simulink model "IEEE34bus_v2019b_Phasor_PI_ZIPload"  (R2024a)
settings: Solver=ode4  StartTime=0.0  StopTime=100  FixedStep=Ts  MaxStep=1e-4  RelTol=1e-4
InitFcn:
  | a=1; % Loading Factor
  | Ts=0.1;% For Delay Blocks in Voltage Regulator Controls
  | % phase to sequence conversion of RXB matrices
  | c=1*exp(sqrt(-1)*(120*pi/180));
  | T=[1 1 1;1 c*c c;1 c c*c];
  | Tinv=1/3*[1 1 1;1 c c*c;1 c*c c];
  | 
  | % Simulation data for the IEEE 34 Node Test Feeder model
  | mi2km = 1.60934;%  miles to km conversion
  | ft2km = 0.0003048; % feet to km conversion
  | ms2F = 1*1e-6/(2*pi*60);% microsiemens to Farads conversion
  | 
  | %% Configuration 300 - series reactance - ohm/mile
  | R_300 = [1.3368 0.2101 0.2130;0.2101 1.3238 0.2066;0.2130 0.2066 1.3294];
  | X_300 = [1.3343 0.5779 0.5015;0.5779 1.3569 0.4591;0.5015 0.4591 1.3471];
  | % charging susceptance - microsiemens/mile
  | B_300 = [5.3350 -1.5313 -0.9943;-1.5313 5.0979 -0.6212;-0.9943 -0.6212 4.8880];
  | 
  | R_300 = R_300/mi2km;
  | Rseq=Tinv*R_300*T;
  | R1_300=Rseq(2,2);R0_300=Rseq(1,1);
  | 
  | L_300 = (X_300/(2*pi*60))/mi2km;
  | Lseq=Tinv*L_300*T;
  | L1_300=Lseq(2,2);L0_300=Lseq(1,1);
  | 
  | C_300 =(B_300*ms2F)/mi2km;
  | Cseq=Tinv*C_300*T;
  | C1_300=Cseq(2,2);C0_300=Cseq(1,1);
  | 
  | %% Configuration 301 - series reactance - ohm/mile
  | R_301 = [1.9300 0.2327 0.2359;0.2327 1.9157 0.2288;0.2359 0.2288 1.9219];
  | X_301 = [1.4115 0.6442 0.5691;0.6442 1.4281 0.5238;0.5691 0.5238 1.4209];
  | % charging susceptance - microsiemens/mile
  | B_301 = [5.1207 -1.4364 -0.9402;-1.4364 4.9055 -0.5951;-0.9402 -0.5951 4.7154];
  | 
  | R_301 = R_301/mi2km;
  | Rseq=Tinv*R_301*T;
  | R1_301=Rseq(2,2);R0_301=Rseq(1,1);
  | 
  | L_301 = (X_301/(2*pi*60))/mi2km;
  | Lseq=Tinv*L_301*T;
  | L1_301=Lseq(2,2);L0_301=Lseq(1,1);
  | 
  | C_301 =(B_301*ms2F)/mi2km;
  | Cseq=Tinv*C_301*T;
  | C1_301=Cseq(2,2);C0_301=Cseq(1,1);
  | 
  | %% Configuration 302 - series reactance - ohm/mile
  | R_302 = [2.7995 0 0;0 0 0;0 0 0];
  | X_302 = [1.4855 0 0;0 0 0;0 0 0];
  | % charging susceptance - microsiemens/mile
  | B_302 = [4.2251 0 0;0 0 0;0 0 0];
  | 
  | R_302 = R_302/mi2km;
  | Rseq=Tinv*R_302*T;
  | R1_302=Rseq(2,2);R0_302=Rseq(1,1);
  | 
  | L_302 = (X_302/(2*pi*60))/mi2km;
  | Lseq=Tinv*L_302*T;
  | ... (+41 lines)
undefined symbols (not defined in the file): find_system, j
libraries: spsSeriesRLCBranchLib x157, spsGroundLib x103, spsVoltageMeasurementLib x100, spsControlledCurrentSourceLib x94, spsThreePhaseVIMeasurementLib x37, spsThreePhasePISectionLineLib x20, spsCurrentMeasurementLib x12, spsOnDelayLib x12, spsPiSectionLineLib x8, spsControlledVoltageSourceLib x6, spsDiscreteVariableTimeDelayLib x6, spsMutualInductanceLib x4
(part 7 of 8)

== system IEEE34bus_v2019b_Phasor_PI_ZIPload/Regulator 2/Single Phase SVR_B/Voltage Regulator Control/Tap Changer Control/Edge Detector ==
  note: Edge or Slope Detector
  In : Inport
  Constant1 : Constant  Value=model
  Demux : Demux  Outputs=2
      settings: DisplayOption=none
  Logical Operator1 : Logic  Operator=OR
  Memory : Memory  InitialCondition=ic  LinearizeAsDelay=on
  Multiport Switch : MultiPortSwitch  InputSameDT=off
  NEGATIVE Edge : Subsystem  TreatAsAtomicUnit=on
  POSITIVE Edge : Subsystem  TreatAsAtomicUnit=on
  either edge : Constant  Value=[1 1]
  neg. edge : Constant  Value=[0 1]
  pos. edge : Constant  Value=[1 0]
  Out : Outport  VectorParamsAs1DForOutWhenUnconnected=off
  wires:
  either edge/1 -> Multiport Switch/4
  Demux/2 -> NEGATIVE Edge/Enable
  Demux/1 -> POSITIVE Edge/Enable
  Multiport Switch/1 -> Demux/1
  Constant1/1 -> Multiport Switch/1
  neg. edge/1 -> Multiport Switch/3
  pos. edge/1 -> Multiport Switch/2
  In/1 -> Memory/1, NEGATIVE Edge/1(IN), POSITIVE Edge/1(IN)
  Memory/1 -> NEGATIVE Edge/2(IN previous), POSITIVE Edge/2(IN previous)
  POSITIVE Edge/1(OUT) -> Logical Operator1/1
  NEGATIVE Edge/1(OUT) -> Logical Operator1/2
  Logical Operator1/1 -> Out/1

== system IEEE34bus_v2019b_Phasor_PI_ZIPload/Regulator 2/Single Phase SVR_C/Voltage Regulator Control/Tap Changer Control/Determine tap position ==
  NewTap : Inport
  Trigger : TriggerPort  VariantControl=Variant
  Memory : Memory  InitialCondition=InitialPosition  InheritSampleTime=on
  Saturation : Saturate  UpperLimit=MinMaxTap(2)  LowerLimit=MinMaxTap(1)
  Sum : Sum  Inputs=|++  SaturateOnIntegerOverflow=on
  TapNo : Outport  InitialOutput=InitialPosition  VectorParamsAs1DForOutWhenUnconnected=off
  wires:
  NewTap/1 -> Sum/1
  Sum/1 -> Saturation/1
  Memory/1 -> Sum/2
  Saturation/1 -> TapNo/1, Memory/1

== system IEEE34bus_v2019b_Phasor_PI_ZIPload/Regulator 2/Single Phase SVR_C/Voltage Regulator Control/Tap Changer Control/Edge Detector ==
  note: Edge or Slope Detector
  In : Inport
  Constant1 : Constant  Value=model
  Demux : Demux  Outputs=2
      settings: DisplayOption=none
  Logical Operator1 : Logic  Operator=OR
  Memory : Memory  InitialCondition=ic  LinearizeAsDelay=on
  Multiport Switch : MultiPortSwitch  InputSameDT=off
  NEGATIVE Edge : Subsystem  TreatAsAtomicUnit=on
  POSITIVE Edge : Subsystem  TreatAsAtomicUnit=on
  either edge : Constant  Value=[1 1]
  neg. edge : Constant  Value=[0 1]
  pos. edge : Constant  Value=[1 0]
  Out : Outport  VectorParamsAs1DForOutWhenUnconnected=off
  wires:
  either edge/1 -> Multiport Switch/4
  Demux/2 -> NEGATIVE Edge/Enable
  Demux/1 -> POSITIVE Edge/Enable
  Multiport Switch/1 -> Demux/1
  Constant1/1 -> Multiport Switch/1
  neg. edge/1 -> Multiport Switch/3
  pos. edge/1 -> Multiport Switch/2
  In/1 -> Memory/1, NEGATIVE Edge/1(IN), POSITIVE Edge/1(IN)
  Memory/1 -> NEGATIVE Edge/2(IN previous), POSITIVE Edge/2(IN previous)
  POSITIVE Edge/1(OUT) -> Logical Operator1/1
  NEGATIVE Edge/1(OUT) -> Logical Operator1/2
  Logical Operator1/1 -> Out/1

== system IEEE34bus_v2019b_Phasor_PI_ZIPload/Regulator 1/Single Phase SVR_A/Voltage Regulator Control/Tap Changer Control/Edge Detector/NEGATIVE Edge ==
  IN : Inport
  IN previous : Inport  Port=2
  Enable : EnablePort  PropagateVarSize=During execution
  Relational Operator1 : RelationalOperator  Operator=>
  OUT : Outport  VectorParamsAs1DForOutWhenUnconnected=off
  wires:
  IN/1 -> Relational Operator1/2
  IN previous/1 -> Relational Operator1/1
  Relational Operator1/1 -> OUT/1

== system IEEE34bus_v2019b_Phasor_PI_ZIPload/Regulator 1/Single Phase SVR_A/Voltage Regulator Control/Tap Changer Control/Edge Detector/POSITIVE Edge ==
  IN : Inport
  IN previous : Inport  Port=2
  Enable : EnablePort  PropagateVarSize=During execution
  Relational Operator1 : RelationalOperator  Operator=>
  OUT : Outport  VectorParamsAs1DForOutWhenUnconnected=off
  wires:
  IN/1 -> Relational Operator1/1
  IN previous/1 -> Relational Operator1/2
  Relational Operator1/1 -> OUT/1

== system IEEE34bus_v2019b_Phasor_PI_ZIPload/Regulator 1/Single Phase SVR_B/Voltage Regulator Control/Tap Changer Control/Edge Detector/NEGATIVE Edge ==
  IN : Inport
  IN previous : Inport  Port=2
  Enable : EnablePort  PropagateVarSize=During execution
  Relational Operator1 : RelationalOperator  Operator=>
  OUT : Outport  VectorParamsAs1DForOutWhenUnconnected=off
  wires:
  IN/1 -> Relational Operator1/2
  IN previous/1 -> Relational Operator1/1
  Relational Operator1/1 -> OUT/1

== system IEEE34bus_v2019b_Phasor_PI_ZIPload/Regulator 1/Single Phase SVR_B/Voltage Regulator Control/Tap Changer Control/Edge Detector/POSITIVE Edge ==
  IN : Inport
  IN previous : Inport  Port=2
  Enable : EnablePort  PropagateVarSize=During execution
  Relational Operator1 : RelationalOperator  Operator=>
  OUT : Outport  VectorParamsAs1DForOutWhenUnconnected=off
  wires:
  IN/1 -> Relational Operator1/1
  IN previous/1 -> Relational Operator1/2
  Relational Operator1/1 -> OUT/1

== system IEEE34bus_v2019b_Phasor_PI_ZIPload/Regulator 1/Single Phase SVR_C/Voltage Regulator Control/Tap Changer Control/Edge Detector/NEGATIVE Edge ==
  IN : Inport
  IN previous : Inport  Port=2
  Enable : EnablePort  PropagateVarSize=During execution
  Relational Operator1 : RelationalOperator  Operator=>
  OUT : Outport  VectorParamsAs1DForOutWhenUnconnected=off
  wires:
  IN/1 -> Relational Operator1/2
  IN previous/1 -> Relational Operator1/1
  Relational Operator1/1 -> OUT/1

== system IEEE34bus_v2019b_Phasor_PI_ZIPload/Regulator 1/Single Phase SVR_C/Voltage Regulator Control/Tap Changer Control/Edge Detector/POSITIVE Edge ==
  IN : Inport
  IN previous : Inport  Port=2
  Enable : EnablePort  PropagateVarSize=During execution
  Relational Operator1 : RelationalOperator  Operator=>
  OUT : Outport  VectorParamsAs1DForOutWhenUnconnected=off
  wires:
  IN/1 -> Relational Operator1/1
  IN previous/1 -> Relational Operator1/2
  Relational Operator1/1 -> OUT/1

== system IEEE34bus_v2019b_Phasor_PI_ZIPload/Regulator 2/Single Phase SVR_A/Voltage Regulator Control/Tap Changer Control/Edge Detector/NEGATIVE Edge ==
  IN : Inport
  IN previous : Inport  Port=2
  Enable : EnablePort  PropagateVarSize=During execution
  Relational Operator1 : RelationalOperator  Operator=>
  OUT : Outport  VectorParamsAs1DForOutWhenUnconnected=off
  wires:
  IN/1 -> Relational Operator1/2
  IN previous/1 -> Relational Operator1/1
  Relational Operator1/1 -> OUT/1

== system IEEE34bus_v2019b_Phasor_PI_ZIPload/Regulator 2/Single Phase SVR_A/Voltage Regulator Control/Tap Changer Control/Edge Detector/POSITIVE Edge ==
  IN : Inport
  IN previous : Inport  Port=2
  Enable : EnablePort  PropagateVarSize=During execution
  Relational Operator1 : RelationalOperator  Operator=>
  OUT : Outport  VectorParamsAs1DForOutWhenUnconnected=off
  wires:
  IN/1 -> Relational Operator1/1
  IN previous/1 -> Relational Operator1/2
  Relational Operator1/1 -> OUT/1

== system IEEE34bus_v2019b_Phasor_PI_ZIPload/Regulator 2/Single Phase SVR_B/Voltage Regulator Control/Tap Changer Control/Edge Detector/NEGATIVE Edge ==
  IN : Inport
  IN previous : Inport  Port=2
  Enable : EnablePort  PropagateVarSize=During execution
  Relational Operator1 : RelationalOperator  Operator=>
  OUT : Outport  VectorParamsAs1DForOutWhenUnconnected=off
  wires:
  IN/1 -> Relational Operator1/2
  IN previous/1 -> Relational Operator1/1
  Relational Operator1/1 -> OUT/1

== system IEEE34bus_v2019b_Phasor_PI_ZIPload/Regulator 2/Single Phase SVR_B/Voltage Regulator Control/Tap Changer Control/Edge Detector/POSITIVE Edge ==
  IN : Inport
  IN previous : Inport  Port=2
  Enable : EnablePort  PropagateVarSize=During execution
  Relational Operator1 : RelationalOperator  Operator=>
  OUT : Outport  VectorParamsAs1DForOutWhenUnconnected=off
  wires:
  IN/1 -> Relational Operator1/1
  IN previous/1 -> Relational Operator1/2
  Relational Operator1/1 -> OUT/1

== system IEEE34bus_v2019b_Phasor_PI_ZIPload/Regulator 2/Single Phase SVR_C/Voltage Regulator Control/Tap Changer Control/Edge Detector/NEGATIVE Edge ==
  IN : Inport
  IN previous : Inport  Port=2
  Enable : EnablePort  PropagateVarSize=During execution
  Relational Operator1 : RelationalOperator  Operator=>
  OUT : Outport  VectorParamsAs1DForOutWhenUnconnected=off
  wires:
  IN/1 -> Relational Operator1/2
  IN previous/1 -> Relational Operator1/1
  Relational Operator1/1 -> OUT/1

== system IEEE34bus_v2019b_Phasor_PI_ZIPload/Regulator 2/Single Phase SVR_C/Voltage Regulator Control/Tap Changer Control/Edge Detector/POSITIVE Edge ==
  IN : Inport
  IN previous : Inport  Port=2
  Enable : EnablePort  PropagateVarSize=During execution
  Relational Operator1 : RelationalOperator  Operator=>
  OUT : Outport  VectorParamsAs1DForOutWhenUnconnected=off
  wires:
  IN/1 -> Relational Operator1/1
  IN previous/1 -> Relational Operator1/2
  Relational Operator1/1 -> OUT/1

== matlab function IEEE34bus_v2019b_Phasor_PI_ZIPload/830 Y PQ/Embedded MATLAB Function ==
  data: Iinj output; Vmeas input; LoadType parameter; Vnom parameter; Pnom parameter; Qnom parameter; Vlim parameter
%Single Phase ZIP Load
%Author: Arun Suresh, University of North Carolina, Charlotte
%Iinj=((Pnom+jQnom)/Vmeas)'
function Iinj = InjectedCurrent(Vmeas,LoadType,Vnom,Pnom,Qnom,Vlim)
% Calculate Pl and Ql.
Kz=0;Ki=0;Kp=0;
Vk=(abs(Vmeas)/Vnom);%(Vmeas/Vnom)
switch LoadType  % 1 for Constant Z, 2 for Constant I and 3 for Constant P, 
    case 1
        Kz=1;
    case 2
        if Vk >= Vlim % convert to Constant Z load due to voltage violation
            Ki=1;
        else
            Kz=1;
        end
    case 3
        if Vk >= Vlim % convert to Constant Z load due to voltage violation
           Kp=1;
        else
            Kz=1;
        end          
 
end
Pl=Pnom *((Kz*Vk*Vk)+(Ki*Vk)+(Kp));
Ql=Qnom *((Kz*Vk*Vk)+(Ki*Vk)+(Kp));
% Net Injected Curent.
% j=sqrt(-1);
Iinj = conj((Pl+j*Ql)/Vmeas);

== matlab function IEEE34bus_v2019b_Phasor_PI_ZIPload/830 D Z/Embedded MATLAB Function2 ==
  data: Iinj output; Vmeas input; LoadType parameter; Vnom parameter; Pnom parameter; Qnom parameter; Vlim parameter
%Three Phase Delta ZIP Load
%Author: Arun Suresh, University of North Carolina, Charlotte
%Pl=Pnom(Kz*(Vmeas/Vnom)^2+Ki(Vmeas/Vnom)+Kp), nom-nominal value,meas-measured value
%Ql=Qnom(Kz*(Vmeas/Vnom)^2+Ki(Vmeas/Vnom)+Kp), nom-nominal value,meas-measured value
%Iinj=((Pl+jQl)/Vmeas)'
function Iinj = InjectedCurrent(Vmeas,LoadType,Vnom,Pnom,Qnom,Vlim)
% % Calculate Pl and Ql.
Kz=0;Ki=0;Kp=0;
Vk=(abs(Vmeas)/(Vnom));%(Vmeas/Vnom)
switch LoadType  % 1 for Constant Z, 2 for Constant I and 3 for Constant P, 
    case 1
        Kz=1;
    case 2
        if Vk >= Vlim % convert to Constant Z load due to voltage violation
            Ki=1;
        else
            Kz=1;
        end
    case 3
        if Vk >= Vlim % convert to Constant Z load due to voltage violation
           Kp=1;
        else
            Kz=1;
        end          
 
end
Pl=Pnom'.*((Kz*Vk.*Vk)+(Ki*Vk)+(Kp));
Ql=Qnom'.*((Kz*Vk.*Vk)+(Ki*Vk)+(Kp));
% Net Injected Curent.
% j=sqrt(-1);
Iinj = conj((Pl+j*Ql)./Vmeas);

== matlab function IEEE34bus_v2019b_Phasor_PI_ZIPload/832 D Z/Embedded MATLAB Function2 ==
  data: Iinj output; Vmeas input; LoadType parameter; Vnom parameter; Pnom parameter; Qnom parameter; Vlim parameter
%Three Phase Delta ZIP Load
%Author: Arun Suresh, University of North Carolina, Charlotte
%Pl=Pnom(Kz*(Vmeas/Vnom)^2+Ki(Vmeas/Vnom)+Kp), nom-nominal value,meas-measured value
%Ql=Qnom(Kz*(Vmeas/Vnom)^2+Ki(Vmeas/Vnom)+Kp), nom-nominal value,meas-measured value
%Iinj=((Pl+jQl)/Vmeas)'
function Iinj = InjectedCurrent(Vmeas,LoadType,Vnom,Pnom,Qnom,Vlim)
% % Calculate Pl and Ql.
Kz=0;Ki=0;Kp=0;
Vk=(abs(Vmeas)/(Vnom));%(Vmeas/Vnom)
switch LoadType  % 1 for Constant Z, 2 for Constant I and 3 for Constant P, 
    case 1
        Kz=1;
    case 2
        if Vk >= Vlim % convert to Constant Z load due to voltage violation
            Ki=1;
        else
            Kz=1;
        end
    case 3
        if Vk >= Vlim % convert to Constant Z load due to voltage violation
           Kp=1;
        else
            Kz=1;
        end          
 
end
Pl=Pnom'.*((Kz*Vk.*Vk)+(Ki*Vk)+(Kp));
Ql=Qnom'.*((Kz*Vk.*Vk)+(Ki*Vk)+(Kp));
% Net Injected Curent.
% j=sqrt(-1);
Iinj = conj((Pl+j*Ql)./Vmeas);

== matlab function IEEE34bus_v2019b_Phasor_PI_ZIPload/858 D Z/Embedded MATLAB Function2 ==
  data: Iinj output; Vmeas input; LoadType parameter; Vnom parameter; Pnom parameter; Qnom parameter; Vlim parameter
%Three Phase Delta ZIP Load
%Author: Arun Suresh, University of North Carolina, Charlotte
%Pl=Pnom(Kz*(Vmeas/Vnom)^2+Ki(Vmeas/Vnom)+Kp), nom-nominal value,meas-measured value
%Ql=Qnom(Kz*(Vmeas/Vnom)^2+Ki(Vmeas/Vnom)+Kp), nom-nominal value,meas-measured value
%Iinj=((Pl+jQl)/Vmeas)'
function Iinj = InjectedCurrent(Vmeas,LoadType,Vnom,Pnom,Qnom,Vlim)
% % Calculate Pl and Ql.
Kz=0;Ki=0;Kp=0;
Vk=(abs(Vmeas)/(Vnom));%(Vmeas/Vnom)
switch LoadType  % 1 for Constant Z, 2 for Constant I and 3 for Constant P, 
    case 1
        Kz=1;
    case 2
        if Vk >= Vlim % convert to Constant Z load due to voltage violation
            Ki=1;
        else
            Kz=1;
        end
    case 3
        if Vk >= Vlim % convert to Constant Z load due to voltage violation
           Kp=1;
        else
            Kz=1;
        end          
 
end
Pl=Pnom'.*((Kz*Vk.*Vk)+(Ki*Vk)+(Kp));
Ql=Qnom'.*((Kz*Vk.*Vk)+(Ki*Vk)+(Kp));
% Net Injected Curent.
% j=sqrt(-1);
Iinj = conj((Pl+j*Ql)./Vmeas);

== matlab function IEEE34bus_v2019b_Phasor_PI_ZIPload/858 D PQ/Embedded MATLAB Function2 ==
  data: Iinj output; Vmeas input; LoadType parameter; Vnom parameter; Pnom parameter; Qnom parameter; Vlim parameter
%Three Phase Delta ZIP Load
%Author: Arun Suresh, University of North Carolina, Charlotte
%Pl=Pnom(Kz*(Vmeas/Vnom)^2+Ki(Vmeas/Vnom)+Kp), nom-nominal value,meas-measured value
%Ql=Qnom(Kz*(Vmeas/Vnom)^2+Ki(Vmeas/Vnom)+Kp), nom-nominal value,meas-measured value
%Iinj=((Pl+jQl)/Vmeas)'
function Iinj = InjectedCurrent(Vmeas,LoadType,Vnom,Pnom,Qnom,Vlim)
% % Calculate Pl and Ql.
Kz=0;Ki=0;Kp=0;
Vk=(abs(Vmeas)/(Vnom));%(Vmeas/Vnom)
switch LoadType  % 1 for Constant Z, 2 for Constant I and 3 for Constant P, 
    case 1
        Kz=1;
    case 2
        if Vk >= Vlim % convert to Constant Z load due to voltage violation
            Ki=1;
        else
            Kz=1;
        end
    case 3
        if Vk >= Vlim % convert to Constant Z load due to voltage violation
           Kp=1;
        else
            Kz=1;
        end          
 
end
Pl=Pnom'.*((Kz*Vk.*Vk)+(Ki*Vk)+(Kp));
Ql=Qnom'.*((Kz*Vk.*Vk)+(Ki*Vk)+(Kp));
% Net Injected Curent.
% j=sqrt(-1);
Iinj = conj((Pl+j*Ql)./Vmeas);

== matlab function IEEE34bus_v2019b_Phasor_PI_ZIPload/834 D PQ/Embedded MATLAB Function2 ==
  data: Iinj output; Vmeas input; LoadType parameter; Vnom parameter; Pnom parameter; Qnom parameter; Vlim parameter
%Three Phase Delta ZIP Load
%Author: Arun Suresh, University of North Carolina, Charlotte
%Pl=Pnom(Kz*(Vmeas/Vnom)^2+Ki(Vmeas/Vnom)+Kp), nom-nominal value,meas-measured value
%Ql=Qnom(Kz*(Vmeas/Vnom)^2+Ki(Vmeas/Vnom)+Kp), nom-nominal value,meas-measured value
%Iinj=((Pl+jQl)/Vmeas)'
function Iinj = InjectedCurrent(Vmeas,LoadType,Vnom,Pnom,Qnom,Vlim)
% % Calculate Pl and Ql.
Kz=0;Ki=0;Kp=0;
Vk=(abs(Vmeas)/(Vnom));%(Vmeas/Vnom)
switch LoadType  % 1 for Constant Z, 2 for Constant I and 3 for Constant P, 
    case 1
        Kz=1;
    case 2
        if Vk >= Vlim % convert to Constant Z load due to voltage violation
            Ki=1;
        else
            Kz=1;
        end
    case 3
        if Vk >= Vlim % convert to Constant Z load due to voltage violation
           Kp=1;
        else
            Kz=1;
        end          
 
end
Pl=Pnom'.*((Kz*Vk.*Vk)+(Ki*Vk)+(Kp));
Ql=Qnom'.*((Kz*Vk.*Vk)+(Ki*Vk)+(Kp));
% Net Injected Curent.
% j=sqrt(-1);
Iinj = conj((Pl+j*Ql)./Vmeas);

== matlab function IEEE34bus_v2019b_Phasor_PI_ZIPload/860 D Z/Embedded MATLAB Function2 ==
  data: Iinj output; Vmeas input; LoadType parameter; Vnom parameter; Pnom parameter; Qnom parameter; Vlim parameter
%Three Phase Delta ZIP Load
%Author: Arun Suresh, University of North Carolina, Charlotte
%Pl=Pnom(Kz*(Vmeas/Vnom)^2+Ki(Vmeas/Vnom)+Kp), nom-nominal value,meas-measured value
%Ql=Qnom(Kz*(Vmeas/Vnom)^2+Ki(Vmeas/Vnom)+Kp), nom-nominal value,meas-measured value
%Iinj=((Pl+jQl)/Vmeas)'
function Iinj = InjectedCurrent(Vmeas,LoadType,Vnom,Pnom,Qnom,Vlim)
% % Calculate Pl and Ql.
Kz=0;Ki=0;Kp=0;
Vk=(abs(Vmeas)/(Vnom));%(Vmeas/Vnom)
switch LoadType  % 1 for Constant Z, 2 for Constant I and 3 for Constant P, 
    case 1
        Kz=1;
    case 2
        if Vk >= Vlim % convert to Constant Z load due to voltage violation
            Ki=1;
        else
            Kz=1;
        end
    case 3
        if Vk >= Vlim % convert to Constant Z load due to voltage violation
           Kp=1;
        else
            Kz=1;
        end          
 
end
Pl=Pnom'.*((Kz*Vk.*Vk)+(Ki*Vk)+(Kp));
Ql=Qnom'.*((Kz*Vk.*Vk)+(Ki*Vk)+(Kp));
% Net Injected Curent.
% j=sqrt(-1);
Iinj = conj((Pl+j*Ql)./Vmeas);

== matlab function IEEE34bus_v2019b_Phasor_PI_ZIPload/834 D Z/Embedded MATLAB Function2 ==
  data: Iinj output; Vmeas input; LoadType parameter; Vnom parameter; Pnom parameter; Qnom parameter; Vlim parameter
%Three Phase Delta ZIP Load
%Author: Arun Suresh, University of North Carolina, Charlotte
%Pl=Pnom(Kz*(Vmeas/Vnom)^2+Ki(Vmeas/Vnom)+Kp), nom-nominal value,meas-measured value
%Ql=Qnom(Kz*(Vmeas/Vnom)^2+Ki(Vmeas/Vnom)+Kp), nom-nominal value,meas-measured value
%Iinj=((Pl+jQl)/Vmeas)'
function Iinj = InjectedCurrent(Vmeas,LoadType,Vnom,Pnom,Qnom,Vlim)
% % Calculate Pl and Ql.
Kz=0;Ki=0;Kp=0;
Vk=(abs(Vmeas)/(Vnom));%(Vmeas/Vnom)
switch LoadType  % 1 for Constant Z, 2 for Constant I and 3 for Constant P, 
    case 1
        Kz=1;
    case 2
        if Vk >= Vlim % convert to Constant Z load due to voltage violation
            Ki=1;
        else
            Kz=1;
        end
    case 3
        if Vk >= Vlim % convert to Constant Z load due to voltage violation
           Kp=1;
        else
            Kz=1;
        end          
 
end
Pl=Pnom'.*((Kz*Vk.*Vk)+(Ki*Vk)+(Kp));
Ql=Qnom'.*((Kz*Vk.*Vk)+(Ki*Vk)+(Kp));
% Net Injected Curent.
% j=sqrt(-1);
Iinj = conj((Pl+j*Ql)./Vmeas);

== matlab function IEEE34bus_v2019b_Phasor_PI_ZIPload/890 D I/Embedded MATLAB Function2 ==
  data: Iinj output; Vmeas input; LoadType parameter; Vnom parameter; Pnom parameter; Qnom parameter; Vlim parameter
%Three Phase Delta ZIP Load
%Author: Arun Suresh, University of North Carolina, Charlotte
%Pl=Pnom(Kz*(Vmeas/Vnom)^2+Ki(Vmeas/Vnom)+Kp), nom-nominal value,meas-measured value
%Ql=Qnom(Kz*(Vmeas/Vnom)^2+Ki(Vmeas/Vnom)+Kp), nom-nominal value,meas-measured value
%Iinj=((Pl+jQl)/Vmeas)'
function Iinj = InjectedCurrent(Vmeas,LoadType,Vnom,Pnom,Qnom,Vlim)
% % Calculate Pl and Ql.
Kz=0;Ki=0;Kp=0;
Vk=(abs(Vmeas)/(Vnom));%(Vmeas/Vnom)
switch LoadType  % 1 for Constant Z, 2 for Constant I and 3 for Constant P, 
    case 1
        Kz=1;
    case 2
        if Vk >= Vlim % convert to Constant Z load due to voltage violation
            Ki=1;
        else
            Kz=1;
        end
    case 3
        if Vk >= Vlim % convert to Constant Z load due to voltage violation
           Kp=1;
        else
            Kz=1;
        end          
 
end
Pl=Pnom'.*((Kz*Vk.*Vk)+(Ki*Vk)+(Kp));
Ql=Qnom'.*((Kz*Vk.*Vk)+(Ki*Vk)+(Kp));
% Net Injected Curent.
% j=sqrt(-1);
Iinj = conj((Pl+j*Ql)./Vmeas);

== matlab function IEEE34bus_v2019b_Phasor_PI_ZIPload/860 D PQ/Embedded MATLAB Function2 ==
  data: Iinj output; Vmeas input; LoadType parameter; Vnom parameter; Pnom parameter; Qnom parameter; Vlim parameter
%Three Phase Delta ZIP Load
%Author: Arun Suresh, University of North Carolina, Charlotte
%Pl=Pnom(Kz*(Vmeas/Vnom)^2+Ki(Vmeas/Vnom)+Kp), nom-nominal value,meas-measured value
%Ql=Qnom(Kz*(Vmeas/Vnom)^2+Ki(Vmeas/Vnom)+Kp), nom-nominal value,meas-measured value
%Iinj=((Pl+jQl)/Vmeas)'
function Iinj = InjectedCurrent(Vmeas,LoadType,Vnom,Pnom,Qnom,Vlim)
% % Calculate Pl and Ql.
Kz=0;Ki=0;Kp=0;
Vk=(abs(Vmeas)/(Vnom));%(Vmeas/Vnom)
switch LoadType  % 1 for Constant Z, 2 for Constant I and 3 for Constant P, 
    case 1
        Kz=1;
    case 2
        if Vk >= Vlim % convert to Constant Z load due to voltage violation
            Ki=1;
        else
            Kz=1;
        end
    case 3
        if Vk >= Vlim % convert to Constant Z load due to voltage violation
           Kp=1;
        else
            Kz=1;
        end          
 
end
Pl=Pnom'.*((Kz*Vk.*Vk)+(Ki*Vk)+(Kp));
Ql=Qnom'.*((Kz*Vk.*Vk)+(Ki*Vk)+(Kp));
% Net Injected Curent.
% j=sqrt(-1);
Iinj = conj((Pl+j*Ql)./Vmeas);

== matlab function IEEE34bus_v2019b_Phasor_PI_ZIPload/860 Y PQ/Embedded MATLAB Function2 ==
  data: Iinj output; Vmeas input; LoadType parameter; Vnom parameter; Pnom parameter; Qnom parameter; Vlim parameter
%Three Phase Star ZIP Load
%Author: Arun Suresh, University of North Carolina, Charlotte
%Pl=Pnom(Kz*(Vmeas/Vnom)^2+Ki(Vmeas/Vnom)+Kp), nom-nominal value,meas-measured value
%Ql=Qnom(Kz*(Vmeas/Vnom)^2+Ki(Vmeas/Vnom)+Kp), nom-nominal value,meas-measured value
%Iinj=((Pl+jQl)/Vmeas)'
function Iinj = InjectedCurrent(Vmeas,LoadType,Vnom,Pnom,Qnom,Vlim)
% % Calculate Pl and Ql.
Kz=0;Ki=0;Kp=0;
Vk=(abs(Vmeas)/(Vnom/sqrt(3)));%(Vmeas/Vnom)
switch LoadType  % 1 for Constant Z, 2 for Constant I and 3 for Constant P, 
    case 1
        Kz=1;
    case 2
        if Vk >= Vlim % convert to Constant Z load due to voltage violation
            Ki=1;
        else
            Kz=1;
        end
    case 3
        if Vk >= Vlim % convert to Constant Z load due to voltage violation
           Kp=1;
        else
            Kz=1;
        end          
 
end
Pl=Pnom'.*((Kz*Vk.*Vk)+(Ki*Vk)+(Kp));
Ql=Qnom'.*((Kz*Vk.*Vk)+(Ki*Vk)+(Kp));
% Net Injected Curent.
Iinj = conj((Pl+j*Ql)./Vmeas);

== matlab function IEEE34bus_v2019b_Phasor_PI_ZIPload/836 D PQ/Embedded MATLAB Function2 ==
  data: Iinj output; Vmeas input; LoadType parameter; Vnom parameter; Pnom parameter; Qnom parameter; Vlim parameter
%Three Phase Delta ZIP Load
%Author: Arun Suresh, University of North Carolina, Charlotte
%Pl=Pnom(Kz*(Vmeas/Vnom)^2+Ki(Vmeas/Vnom)+Kp), nom-nominal value,meas-measured value
%Ql=Qnom(Kz*(Vmeas/Vnom)^2+Ki(Vmeas/Vnom)+Kp), nom-nominal value,meas-measured value
%Iinj=((Pl+jQl)/Vmeas)'
function Iinj = InjectedCurrent(Vmeas,LoadType,Vnom,Pnom,Qnom,Vlim)
% % Calculate Pl and Ql.
Kz=0;Ki=0;Kp=0;
Vk=(abs(Vmeas)/(Vnom));%(Vmeas/Vnom)
switch LoadType  % 1 for Constant Z, 2 for Constant I and 3 for Constant P, 
    case 1
        Kz=1;
    case 2
        if Vk >= Vlim % convert to Constant Z load due to voltage violation
            Ki=1;
        else
            Kz=1;
        end
    case 3
        if Vk >= Vlim % convert to Constant Z load due to voltage violation
           Kp=1;
        else
            Kz=1;
        end          
 
end
Pl=Pnom'.*((Kz*Vk.*Vk)+(Ki*Vk)+(Kp));
Ql=Qnom'.*((Kz*Vk.*Vk)+(Ki*Vk)+(Kp));
% Net Injected Curent.
% j=sqrt(-1);
Iinj = conj((Pl+j*Ql)./Vmeas);

== matlab function IEEE34bus_v2019b_Phasor_PI_ZIPload/836 D I/Embedded MATLAB Function2 ==
  data: Iinj output; Vmeas input; LoadType parameter; Vnom parameter; Pnom parameter; Qnom parameter; Vlim parameter
%Three Phase Delta ZIP Load
%Author: Arun Suresh, University of North Carolina, Charlotte
%Pl=Pnom(Kz*(Vmeas/Vnom)^2+Ki(Vmeas/Vnom)+Kp), nom-nominal value,meas-measured value
%Ql=Qnom(Kz*(Vmeas/Vnom)^2+Ki(Vmeas/Vnom)+Kp), nom-nominal value,meas-measured value
%Iinj=((Pl+jQl)/Vmeas)'
function Iinj = InjectedCurrent(Vmeas,LoadType,Vnom,Pnom,Qnom,Vlim)
% % Calculate Pl and Ql.
Kz=0;Ki=0;Kp=0;
Vk=(abs(Vmeas)/(Vnom));%(Vmeas/Vnom)
switch LoadType  % 1 for Constant Z, 2 for Constant I and 3 for Constant P, 
    case 1
        Kz=1;
    case 2
        if Vk >= Vlim % convert to Constant Z load due to voltage violation
            Ki=1;
        else
            Kz=1;
        end
    case 3
        if Vk >= Vlim % convert to Constant Z load due to voltage violation
           Kp=1;
        else
            Kz=1;
        end          
 
end
Pl=Pnom'.*((Kz*Vk.*Vk)+(Ki*Vk)+(Kp));
Ql=Qnom'.*((Kz*Vk.*Vk)+(Ki*Vk)+(Kp));
% Net Injected Curent.
% j=sqrt(-1);
Iinj = conj((Pl+j*Ql)./Vmeas);

== matlab function IEEE34bus_v2019b_Phasor_PI_ZIPload/840 D I/Embedded MATLAB Function2 ==
  data: Iinj output; Vmeas input; LoadType parameter; Vnom parameter; Pnom parameter; Qnom parameter; Vlim parameter
%Three Phase Delta ZIP Load
%Author: Arun Suresh, University of North Carolina, Charlotte
%Pl=Pnom(Kz*(Vmeas/Vnom)^2+Ki(Vmeas/Vnom)+Kp), nom-nominal value,meas-measured value
%Ql=Qnom(Kz*(Vmeas/Vnom)^2+Ki(Vmeas/Vnom)+Kp), nom-nominal value,meas-measured value
%Iinj=((Pl+jQl)/Vmeas)'
function Iinj = InjectedCurrent(Vmeas,LoadType,Vnom,Pnom,Qnom,Vlim)
% % Calculate Pl and Ql.
Kz=0;Ki=0;Kp=0;
Vk=(abs(Vmeas)/(Vnom));%(Vmeas/Vnom)
switch LoadType  % 1 for Constant Z, 2 for Constant I and 3 for Constant P, 
    case 1
        Kz=1;
    case 2
        if Vk >= Vlim % convert to Constant Z load due to voltage violation
            Ki=1;
        else
            Kz=1;
        end
    case 3
        if Vk >= Vlim % convert to Constant Z load due to voltage violation
           Kp=1;
        else
            Kz=1;
        end          
 
end
Pl=Pnom'.*((Kz*Vk.*Vk)+(Ki*Vk)+(Kp));
Ql=Qnom'.*((Kz*Vk.*Vk)+(Ki*Vk)+(Kp));
% Net Injected Curent.
% j=sqrt(-1);
Iinj = conj((Pl+j*Ql)./Vmeas);

== matlab function IEEE34bus_v2019b_Phasor_PI_ZIPload/826 Y I1/Embedded MATLAB Function ==
  data: Iinj output; Vmeas input; LoadType parameter; Vnom parameter; Pnom parameter; Qnom parameter; Vlim parameter
%Single Phase ZIP Load
%Author: Arun Suresh, University of North Carolina, Charlotte
%Iinj=((Pnom+jQnom)/Vmeas)'
function Iinj = InjectedCurrent(Vmeas,LoadType,Vnom,Pnom,Qnom,Vlim)
% Calculate Pl and Ql.
Kz=0;Ki=0;Kp=0;
Vk=(abs(Vmeas)/Vnom);%(Vmeas/Vnom)
switch LoadType  % 1 for Constant Z, 2 for Constant I and 3 for Constant P, 
    case 1
        Kz=1;
    case 2
        if Vk >= Vlim % convert to Constant Z load due to voltage violation
            Ki=1;
        else
            Kz=1;
        end
    case 3
        if Vk >= Vlim % convert to Constant Z load due to voltage violation
           Kp=1;
        else
            Kz=1;
        end          
 
end
Pl=Pnom *((Kz*Vk*Vk)+(Ki*Vk)+(Kp));
Ql=Qnom *((Kz*Vk*Vk)+(Ki*Vk)+(Kp));
% Net Injected Curent.
% j=sqrt(-1);
Iinj = conj((Pl+j*Ql)/Vmeas);

== matlab function IEEE34bus_v2019b_Phasor_PI_ZIPload/840 Y I/Embedded MATLAB Function2 ==
  data: Iinj output; Vmeas input; LoadType parameter; Vnom parameter; Pnom parameter; Qnom parameter; Vlim parameter
%Three Phase Star ZIP Load
%Author: Arun Suresh, University of North Carolina, Charlotte
%Pl=Pnom(Kz*(Vmeas/Vnom)^2+Ki(Vmeas/Vnom)+Kp), nom-nominal value,meas-measured value
%Ql=Qnom(Kz*(Vmeas/Vnom)^2+Ki(Vmeas/Vnom)+Kp), nom-nominal value,meas-measured value
%Iinj=((Pl+jQl)/Vmeas)'
function Iinj = InjectedCurrent(Vmeas,LoadType,Vnom,Pnom,Qnom,Vlim)
% % Calculate Pl and Ql.
Kz=0;Ki=0;Kp=0;
Vk=(abs(Vmeas)/(Vnom/sqrt(3)));%(Vmeas/Vnom)
switch LoadType  % 1 for Constant Z, 2 for Constant I and 3 for Constant P, 
    case 1
        Kz=1;
    case 2
        if Vk >= Vlim % convert to Constant Z load due to voltage violation
            Ki=1;
        else
            Kz=1;
        end
    case 3
        if Vk >= Vlim % convert to Constant Z load due to voltage violation
           Kp=1;
        else
            Kz=1;
        end          
 
end
Pl=Pnom'.*((Kz*Vk.*Vk)+(Ki*Vk)+(Kp));
Ql=Qnom'.*((Kz*Vk.*Vk)+(Ki*Vk)+(Kp));
% Net Injected Curent.
Iinj = conj((Pl+j*Ql)./Vmeas);

== matlab function IEEE34bus_v2019b_Phasor_PI_ZIPload/844 Y PQ/Embedded MATLAB Function ==
  data: Iinj output; Vmeas input; LoadType parameter; Vnom parameter; Pnom parameter; Qnom parameter; Vlim parameter
%Single Phase ZIP Load
%Author: Arun Suresh, University of North Carolina, Charlotte
%Iinj=((Pnom+jQnom)/Vmeas)'
function Iinj = InjectedCurrent(Vmeas,LoadType,Vnom,Pnom,Qnom,Vlim)
% Calculate Pl and Ql.
Kz=0;Ki=0;Kp=0;
Vk=(abs(Vmeas)/Vnom);%(Vmeas/Vnom)
switch LoadType  % 1 for Constant Z, 2 for Constant I and 3 for Constant P, 
    case 1
        Kz=1;
    case 2
        if Vk >= Vlim % convert to Constant Z load due to voltage violation
            Ki=1;
        else
            Kz=1;
        end
    case 3
        if Vk >= Vlim % convert to Constant Z load due to voltage violation
           Kp=1;
        else
            Kz=1;
        end          
 
end
Pl=Pnom *((Kz*Vk*Vk)+(Ki*Vk)+(Kp));
Ql=Qnom *((Kz*Vk*Vk)+(Ki*Vk)+(Kp));
% Net Injected Curent.
% j=sqrt(-1);
Iinj = conj((Pl+j*Ql)/Vmeas);

== matlab function IEEE34bus_v2019b_Phasor_PI_ZIPload/842 Y PQ/Embedded MATLAB Function ==
  data: Iinj output; Vmeas input; LoadType parameter; Vnom parameter; Pnom parameter; Qnom parameter; Vlim parameter
%Single Phase ZIP Load
%Author: Arun Suresh, University of North Carolina, Charlotte
%Iinj=((Pnom+jQnom)/Vmeas)'
function Iinj = InjectedCurrent(Vmeas,LoadType,Vnom,Pnom,Qnom,Vlim)
% Calculate Pl and Ql.
Kz=0;Ki=0;Kp=0;
Vk=(abs(Vmeas)/Vnom);%(Vmeas/Vnom)
switch LoadType  % 1 for Constant Z, 2 for Constant I and 3 for Constant P, 
    case 1
        Kz=1;
    case 2
        if Vk >= Vlim % convert to Constant Z load due to voltage violation
            Ki=1;
        else
            Kz=1;
        end
    case 3
        if Vk >= Vlim % convert to Constant Z load due to voltage violation
           Kp=1;
        else
            Kz=1;
        end          
 
end
Pl=Pnom *((Kz*Vk*Vk)+(Ki*Vk)+(Kp));
Ql=Qnom *((Kz*Vk*Vk)+(Ki*Vk)+(Kp));
% Net Injected Curent.
% j=sqrt(-1);
Iinj = conj((Pl+j*Ql)/Vmeas);

== matlab function IEEE34bus_v2019b_Phasor_PI_ZIPload/844 Y Z/Embedded MATLAB Function2 ==
  data: Iinj output; Vmeas input; LoadType parameter; Vnom parameter; Pnom parameter; Qnom parameter; Vlim parameter
%Three Phase Star ZIP Load
%Author: Arun Suresh, University of North Carolina, Charlotte
%Pl=Pnom(Kz*(Vmeas/Vnom)^2+Ki(Vmeas/Vnom)+Kp), nom-nominal value,meas-measured value
%Ql=Qnom(Kz*(Vmeas/Vnom)^2+Ki(Vmeas/Vnom)+Kp), nom-nominal value,meas-measured value
%Iinj=((Pl+jQl)/Vmeas)'
function Iinj = InjectedCurrent(Vmeas,LoadType,Vnom,Pnom,Qnom,Vlim)
% % Calculate Pl and Ql.
Kz=0;Ki=0;Kp=0;
Vk=(abs(Vmeas)/(Vnom/sqrt(3)));%(Vmeas/Vnom)
switch LoadType  % 1 for Constant Z, 2 for Constant I and 3 for Constant P, 
    case 1
        Kz=1;
    case 2
        if Vk >= Vlim % convert to Constant Z load due to voltage violation
            Ki=1;
        else
            Kz=1;
        end
    case 3
        if Vk >= Vlim % convert to Constant Z load due to voltage violation
           Kp=1;
        else
            Kz=1;
        end          
 
end
Pl=Pnom'.*((Kz*Vk.*Vk)+(Ki*Vk)+(Kp));
Ql=Qnom'.*((Kz*Vk.*Vk)+(Ki*Vk)+(Kp));
% Net Injected Curent.
Iinj = conj((Pl+j*Ql)./Vmeas);

== matlab function IEEE34bus_v2019b_Phasor_PI_ZIPload/846 Y PQ/Embedded MATLAB Function2 ==
  data: Iinj output; Vmeas input; LoadType parameter; Vnom parameter; Pnom parameter; Qnom parameter; Vlim parameter
%Three Phase Star ZIP Load
%Author: Arun Suresh, University of North Carolina, Charlotte
%Pl=Pnom(Kz*(Vmeas/Vnom)^2+Ki(Vmeas/Vnom)+Kp), nom-nominal value,meas-measured value
%Ql=Qnom(Kz*(Vmeas/Vnom)^2+Ki(Vmeas/Vnom)+Kp), nom-nominal value,meas-measured value
%Iinj=((Pl+jQl)/Vmeas)'
function Iinj = InjectedCurrent(Vmeas,LoadType,Vnom,Pnom,Qnom,Vlim)
% % Calculate Pl and Ql.
Kz=0;Ki=0;Kp=0;
Vk=(abs(Vmeas)/(Vnom/sqrt(3)));%(Vmeas/Vnom)
switch LoadType  % 1 for Constant Z, 2 for Constant I and 3 for Constant P, 
    case 1
        Kz=1;
    case 2
        if Vk >= Vlim % convert to Constant Z load due to voltage violation
            Ki=1;
        else
            Kz=1;
        end
    case 3
        if Vk >= Vlim % convert to Constant Z load due to voltage violation
           Kp=1;
        else
            Kz=1;
        end          
 
end
Pl=Pnom'.*((Kz*Vk.*Vk)+(Ki*Vk)+(Kp));
Ql=Qnom'.*((Kz*Vk.*Vk)+(Ki*Vk)+(Kp));
% Net Injected Curent.
Iinj = conj((Pl+j*Ql)./Vmeas);

== matlab function IEEE34bus_v2019b_Phasor_PI_ZIPload/844 Y PQ1/Embedded MATLAB Function2 ==
  data: Iinj output; Vmeas input; LoadType parameter; Vnom parameter; Pnom parameter; Qnom parameter; Vlim parameter
%Three Phase Star ZIP Load
%Author: Arun Suresh, University of North Carolina, Charlotte
%Pl=Pnom(Kz*(Vmeas/Vnom)^2+Ki(Vmeas/Vnom)+Kp), nom-nominal value,meas-measured value
%Ql=Qnom(Kz*(Vmeas/Vnom)^2+Ki(Vmeas/Vnom)+Kp), nom-nominal value,meas-measured value
%Iinj=((Pl+jQl)/Vmeas)'
function Iinj = InjectedCurrent(Vmeas,LoadType,Vnom,Pnom,Qnom,Vlim)
% % Calculate Pl and Ql.
Kz=0;Ki=0;Kp=0;
Vk=(abs(Vmeas)/(Vnom/sqrt(3)));%(Vmeas/Vnom)
switch LoadType  % 1 for Constant Z, 2 for Constant I and 3 for Constant P, 
    case 1
        Kz=1;
    case 2
        if Vk >= Vlim % convert to Constant Z load due to voltage violation
            Ki=1;
        else
            Kz=1;
        end
    case 3
        if Vk >= Vlim % convert to Constant Z load due to voltage violation
           Kp=1;
        else
            Kz=1;
        end          
 
end
Pl=Pnom'.*((Kz*Vk.*Vk)+(Ki*Vk)+(Kp));
Ql=Qnom'.*((Kz*Vk.*Vk)+(Ki*Vk)+(Kp));
% Net Injected Curent.
Iinj = conj((Pl+j*Ql)./Vmeas);

== matlab function IEEE34bus_v2019b_Phasor_PI_ZIPload/848 Y PQ/Embedded MATLAB Function ==
  data: Iinj output; Vmeas input; LoadType parameter; Vnom parameter; Pnom parameter; Qnom parameter; Vlim parameter
%Single Phase ZIP Load
%Author: Arun Suresh, University of North Carolina, Charlotte
%Iinj=((Pnom+jQnom)/Vmeas)'
function Iinj = InjectedCurrent(Vmeas,LoadType,Vnom,Pnom,Qnom,Vlim)
% Calculate Pl and Ql.
Kz=0;Ki=0;Kp=0;
Vk=(abs(Vmeas)/Vnom);%(Vmeas/Vnom)
switch LoadType  % 1 for Constant Z, 2 for Constant I and 3 for Constant P, 
    case 1
        Kz=1;
    case 2
        if Vk >= Vlim % convert to Constant Z load due to voltage violation
            Ki=1;
        else
            Kz=1;
        end
    case 3
        if Vk >= Vlim % convert to Constant Z load due to voltage violation
           Kp=1;
        else
            Kz=1;
        end          
 
end
Pl=Pnom *((Kz*Vk*Vk)+(Ki*Vk)+(Kp));
Ql=Qnom *((Kz*Vk*Vk)+(Ki*Vk)+(Kp));
% Net Injected Curent.
% j=sqrt(-1);
Iinj = conj((Pl+j*Ql)/Vmeas);

== matlab function IEEE34bus_v2019b_Phasor_PI_ZIPload/846 Y PQ1/Embedded MATLAB Function ==
  data: Iinj output; Vmeas input; LoadType parameter; Vnom parameter; Pnom parameter; Qnom parameter; Vlim parameter
%Single Phase ZIP Load
%Author: Arun Suresh, University of North Carolina, Charlotte
%Iinj=((Pnom+jQnom)/Vmeas)'
function Iinj = InjectedCurrent(Vmeas,LoadType,Vnom,Pnom,Qnom,Vlim)
% Calculate Pl and Ql.
Kz=0;Ki=0;Kp=0;
Vk=(abs(Vmeas)/Vnom);%(Vmeas/Vnom)
switch LoadType  % 1 for Constant Z, 2 for Constant I and 3 for Constant P, 
    case 1
        Kz=1;
    case 2
        if Vk >= Vlim % convert to Constant Z load due to voltage violation
            Ki=1;
        else
            Kz=1;
        end
    case 3
        if Vk >= Vlim % convert to Constant Z load due to voltage violation
           Kp=1;
        else
            Kz=1;
        end          
 
end
Pl=Pnom *((Kz*Vk*Vk)+(Ki*Vk)+(Kp));
Ql=Qnom *((Kz*Vk*Vk)+(Ki*Vk)+(Kp));
% Net Injected Curent.
% j=sqrt(-1);
Iinj = conj((Pl+j*Ql)/Vmeas);

== matlab function IEEE34bus_v2019b_Phasor_PI_ZIPload/848 D PQ/Embedded MATLAB Function2 ==
  data: Iinj output; Vmeas input; LoadType parameter; Vnom parameter; Pnom parameter; Qnom parameter; Vlim parameter
%Three Phase Delta ZIP Load
%Author: Arun Suresh, University of North Carolina, Charlotte
%Pl=Pnom(Kz*(Vmeas/Vnom)^2+Ki(Vmeas/Vnom)+Kp), nom-nominal value,meas-measured value
%Ql=Qnom(Kz*(Vmeas/Vnom)^2+Ki(Vmeas/Vnom)+Kp), nom-nominal value,meas-measured value
%Iinj=((Pl+jQl)/Vmeas)'
function Iinj = InjectedCurrent(Vmeas,LoadType,Vnom,Pnom,Qnom,Vlim)
% % Calculate Pl and Ql.
Kz=0;Ki=0;Kp=0;
Vk=(abs(Vmeas)/(Vnom));%(Vmeas/Vnom)
switch LoadType  % 1 for Constant Z, 2 for Constant I and 3 for Constant P, 
    case 1
        Kz=1;
    case 2
        if Vk >= Vlim % convert to Constant Z load due to voltage violation
            Ki=1;
        else
            Kz=1;
        end
    case 3
        if Vk >= Vlim % convert to Constant Z load due to voltage violation
           Kp=1;
        else
            Kz=1;
        end          
 
end
Pl=Pnom'.*((Kz*Vk.*Vk)+(Ki*Vk)+(Kp));
Ql=Qnom'.*((Kz*Vk.*Vk)+(Ki*Vk)+(Kp));
% Net Injected Curent.
% j=sqrt(-1);
Iinj = conj((Pl+j*Ql)./Vmeas);

== matlab function IEEE34bus_v2019b_Phasor_PI_ZIPload/862 Y PQ/Embedded MATLAB Function ==
  data: Iinj output; Vmeas input; LoadType parameter; Vnom parameter; Pnom parameter; Qnom parameter; Vlim parameter
%Single Phase ZIP Load
%Author: Arun Suresh, University of North Carolina, Charlotte
%Iinj=((Pnom+jQnom)/Vmeas)'
function Iinj = InjectedCurrent(Vmeas,LoadType,Vnom,Pnom,Qnom,Vlim)
% Calculate Pl and Ql.
Kz=0;Ki=0;Kp=0;
Vk=(abs(Vmeas)/Vnom);%(Vmeas/Vnom)
switch LoadType  % 1 for Constant Z, 2 for Constant I and 3 for Constant P, 
    case 1
        Kz=1;
    case 2
        if Vk >= Vlim % convert to Constant Z load due to voltage violation
            Ki=1;
        else
            Kz=1;
        end
    case 3
        if Vk >= Vlim % convert to Constant Z load due to voltage violation
           Kp=1;
        else
            Kz=1;
        end          
 
end
Pl=Pnom *((Kz*Vk*Vk)+(Ki*Vk)+(Kp));
Ql=Qnom *((Kz*Vk*Vk)+(Ki*Vk)+(Kp));
% Net Injected Curent.
% j=sqrt(-1);
Iinj = conj((Pl+j*Ql)/Vmeas);

== matlab function IEEE34bus_v2019b_Phasor_PI_ZIPload/802 Y PQ/Embedded MATLAB Function2 ==
  data: Iinj output; Vmeas input; LoadType parameter; Vnom parameter; Pnom parameter; Qnom parameter; Vlim parameter
%Three Phase Star ZIP Load
%Author: Arun Suresh, University of North Carolina, Charlotte
%Pl=Pnom(Kz*(Vmeas/Vnom)^2+Ki(Vmeas/Vnom)+Kp), nom-nominal value,meas-measured value
%Ql=Qnom(Kz*(Vmeas/Vnom)^2+Ki(Vmeas/Vnom)+Kp), nom-nominal value,meas-measured value
%Iinj=((Pl+jQl)/Vmeas)'
function Iinj = InjectedCurrent(Vmeas,LoadType,Vnom,Pnom,Qnom,Vlim)
% % Calculate Pl and Ql.
Kz=0;Ki=0;Kp=0;
Vk=(abs(Vmeas)/(Vnom/sqrt(3)));%(Vmeas/Vnom)
switch LoadType  % 1 for Constant Z, 2 for Constant I and 3 for Constant P, 
    case 1
        Kz=1;
    case 2
        if Vk >= Vlim % convert to Constant Z load due to voltage violation
            Ki=1;
        else
            Kz=1;
        end
    case 3
        if Vk >= Vlim % convert to Constant Z load due to voltage violation
           Kp=1;
        else
            Kz=1;
        end          
 
end
Pl=Pnom'.*((Kz*Vk.*Vk)+(Ki*Vk)+(Kp));
Ql=Qnom'.*((Kz*Vk.*Vk)+(Ki*Vk)+(Kp));
% Net Injected Curent.
Iinj = conj((Pl+j*Ql)./Vmeas);

== matlab function IEEE34bus_v2019b_Phasor_PI_ZIPload/838 Y PQ/Embedded MATLAB Function ==
  data: Iinj output; Vmeas input; LoadType parameter; Vnom parameter; Pnom parameter; Qnom parameter; Vlim parameter
%Single Phase ZIP Load
%Author: Arun Suresh, University of North Carolina, Charlotte
%Iinj=((Pnom+jQnom)/Vmeas)'
function Iinj = InjectedCurrent(Vmeas,LoadType,Vnom,Pnom,Qnom,Vlim)
% Calculate Pl and Ql.
Kz=0;Ki=0;Kp=0;
Vk=(abs(Vmeas)/Vnom);%(Vmeas/Vnom)
switch LoadType  % 1 for Constant Z, 2 for Constant I and 3 for Constant P, 
    case 1
        Kz=1;
    case 2
        if Vk >= Vlim % convert to Constant Z load due to voltage violation
            Ki=1;
        else
            Kz=1;
        end
    case 3
        if Vk >= Vlim % convert to Constant Z load due to voltage violation
           Kp=1;
        else
            Kz=1;
        end          
 
end
Pl=Pnom *((Kz*Vk*Vk)+(Ki*Vk)+(Kp));
Ql=Qnom *((Kz*Vk*Vk)+(Ki*Vk)+(Kp));
% Net Injected Curent.
% j=sqrt(-1);
Iinj = conj((Pl+j*Ql)/Vmeas);

== matlab function IEEE34bus_v2019b_Phasor_PI_ZIPload/864 Y PQ/Embedded MATLAB Function ==
  data: Iinj output; Vmeas input; LoadType parameter; Vnom parameter; Pnom parameter; Qnom parameter; Vlim parameter
%Single Phase ZIP Load
%Author: Arun Suresh, University of North Carolina, Charlotte
%Iinj=((Pnom+jQnom)/Vmeas)'
function Iinj = InjectedCurrent(Vmeas,LoadType,Vnom,Pnom,Qnom,Vlim)
% Calculate Pl and Ql.
Kz=0;Ki=0;Kp=0;
Vk=(abs(Vmeas)/Vnom);%(Vmeas/Vnom)
switch LoadType  % 1 for Constant Z, 2 for Constant I and 3 for Constant P, 
    case 1
        Kz=1;
    case 2
        if Vk >= Vlim % convert to Constant Z load due to voltage violation
            Ki=1;
        else
            Kz=1;
        end
    case 3
        if Vk >= Vlim % convert to Constant Z load due to voltage violation
           Kp=1;
        else
            Kz=1;
        end          
 
end
Pl=Pnom *((Kz*Vk*Vk)+(Ki*Vk)+(Kp));
Ql=Qnom *((Kz*Vk*Vk)+(Ki*Vk)+(Kp));
% Net Injected Curent.
% j=sqrt(-1);
Iinj = conj((Pl+j*Ql)/Vmeas);

== matlab function IEEE34bus_v2019b_Phasor_PI_ZIPload/858 Y PQ/Embedded MATLAB Function ==
  data: Iinj output; Vmeas input; LoadType parameter; Vnom parameter; Pnom parameter; Qnom parameter; Vlim parameter
%Single Phase ZIP Load
%Author: Arun Suresh, University of North Carolina, Charlotte
%Iinj=((Pnom+jQnom)/Vmeas)'
function Iinj = InjectedCurrent(Vmeas,LoadType,Vnom,Pnom,Qnom,Vlim)
% Calculate Pl and Ql.
Kz=0;Ki=0;Kp=0;
Vk=(abs(Vmeas)/Vnom);%(Vmeas/Vnom)
switch LoadType  % 1 for Constant Z, 2 for Constant I and 3 for Constant P, 
    case 1
        Kz=1;
    case 2
        if Vk >= Vlim % convert to Constant Z load due to voltage violation
            Ki=1;
        else
            Kz=1;
        end
    case 3
        if Vk >= Vlim % convert to Constant Z load due to voltage violation
           Kp=1;
        else
            Kz=1;
        end          
 
end
Pl=Pnom *((Kz*Vk*Vk)+(Ki*Vk)+(Kp));
Ql=Qnom *((Kz*Vk*Vk)+(Ki*Vk)+(Kp));
% Net Injected Curent.
% j=sqrt(-1);
Iinj = conj((Pl+j*Ql)/Vmeas);

== matlab function IEEE34bus_v2019b_Phasor_PI_ZIPload/854 Y PQ/Embedded MATLAB Function ==
  data: Iinj output; Vmeas input; LoadType parameter; Vnom parameter; Pnom parameter; Qnom parameter; Vlim parameter
%Single Phase ZIP Load
%Author: Arun Suresh, University of North Carolina, Charlotte
%Iinj=((Pnom+jQnom)/Vmeas)'
function Iinj = InjectedCurrent(Vmeas,LoadType,Vnom,Pnom,Qnom,Vlim)
% Calculate Pl and Ql.
Kz=0;Ki=0;Kp=0;
Vk=(abs(Vmeas)/Vnom);%(Vmeas/Vnom)
switch LoadType  % 1 for Constant Z, 2 for Constant I and 3 for Constant P, 
    case 1
        Kz=1;
    case 2
        if Vk >= Vlim % convert to Constant Z load due to voltage violation
            Ki=1;
        else
            Kz=1;
        end
    case 3
        if Vk >= Vlim % convert to Constant Z load due to voltage violation
           Kp=1;
        else
            Kz=1;
        end          
 
end
Pl=Pnom *((Kz*Vk*Vk)+(Ki*Vk)+(Kp));
Ql=Qnom *((Kz*Vk*Vk)+(Ki*Vk)+(Kp));
% Net Injected Curent.
% j=sqrt(-1);
Iinj = conj((Pl+j*Ql)/Vmeas);

== matlab function IEEE34bus_v2019b_Phasor_PI_ZIPload/856 Y PQ/Embedded MATLAB Function ==
  data: Iinj output; Vmeas input; LoadType parameter; Vnom parameter; Pnom parameter; Qnom parameter; Vlim parameter
%Single Phase ZIP Load
%Author: Arun Suresh, University of North Carolina, Charlotte
%Iinj=((Pnom+jQnom)/Vmeas)'
function Iinj = InjectedCurrent(Vmeas,LoadType,Vnom,Pnom,Qnom,Vlim)
% Calculate Pl and Ql.
Kz=0;Ki=0;Kp=0;
Vk=(abs(Vmeas)/Vnom);%(Vmeas/Vnom)
switch LoadType  % 1 for Constant Z, 2 for Constant I and 3 for Constant P, 
    case 1
        Kz=1;
    case 2
        if Vk >= Vlim % convert to Constant Z load due to voltage violation
            Ki=1;
        else
            Kz=1;
        end
    case 3
        if Vk >= Vlim % convert to Constant Z load due to voltage violation
           Kp=1;
        else
            Kz=1;
        end          
 
end
Pl=Pnom *((Kz*Vk*Vk)+(Ki*Vk)+(Kp));
Ql=Qnom *((Kz*Vk*Vk)+(Ki*Vk)+(Kp));
% Net Injected Curent.
% j=sqrt(-1);
Iinj = conj((Pl+j*Ql)/Vmeas);

== matlab function IEEE34bus_v2019b_Phasor_PI_ZIPload/824 Y I/Embedded MATLAB Function ==
  data: Iinj output; Vmeas input; LoadType parameter; Vnom parameter; Pnom parameter; Qnom parameter; Vlim parameter
%Single Phase ZIP Load
%Author: Arun Suresh, University of North Carolina, Charlotte
%Iinj=((Pnom+jQnom)/Vmeas)'
function Iinj = InjectedCurrent(Vmeas,LoadType,Vnom,Pnom,Qnom,Vlim)
% Calculate Pl and Ql.
Kz=0;Ki=0;Kp=0;
Vk=(abs(Vmeas)/Vnom);%(Vmeas/Vnom)
switch LoadType  % 1 for Constant Z, 2 for Constant I and 3 for Constant P, 
    case 1
        Kz=1;
    case 2
        if Vk >= Vlim % convert to Constant Z load due to voltage violation
            Ki=1;
        else
            Kz=1;
        end
    case 3
        if Vk >= Vlim % convert to Constant Z load due to voltage violation
           Kp=1;
        else
            Kz=1;
        end          
 
end
Pl=Pnom *((Kz*Vk*Vk)+(Ki*Vk)+(Kp));
Ql=Qnom *((Kz*Vk*Vk)+(Ki*Vk)+(Kp));
% Net Injected Curent.
% j=sqrt(-1);
Iinj = conj((Pl+j*Ql)/Vmeas);

== matlab function IEEE34bus_v2019b_Phasor_PI_ZIPload/826 Y I/Embedded MATLAB Function ==
  data: Iinj output; Vmeas input; LoadType parameter; Vnom parameter; Pnom parameter; Qnom parameter; Vlim parameter
%Single Phase ZIP Load
%Author: Arun Suresh, University of North Carolina, Charlotte
%Iinj=((Pnom+jQnom)/Vmeas)'
function Iinj = InjectedCurrent(Vmeas,LoadType,Vnom,Pnom,Qnom,Vlim)
% Calculate Pl and Ql.
Kz=0;Ki=0;Kp=0;
Vk=(abs(Vmeas)/Vnom);%(Vmeas/Vnom)
switch LoadType  % 1 for Constant Z, 2 for Constant I and 3 for Constant P, 
    case 1
        Kz=1;
    case 2
        if Vk >= Vlim % convert to Constant Z load due to voltage violation
            Ki=1;
        else
            Kz=1;
        end
    case 3
        if Vk >= Vlim % convert to Constant Z load due to voltage violation
           Kp=1;
        else
            Kz=1;
        end          
 
end
Pl=Pnom *((Kz*Vk*Vk)+(Ki*Vk)+(Kp));
Ql=Qnom *((Kz*Vk*Vk)+(Ki*Vk)+(Kp));
% Net Injected Curent.
% j=sqrt(-1);
Iinj = conj((Pl+j*Ql)/Vmeas);

== matlab function IEEE34bus_v2019b_Phasor_PI_ZIPload/818 Y Z/Embedded MATLAB Function ==
  data: Iinj output; Vmeas input; LoadType parameter; Vnom parameter; Pnom parameter; Qnom parameter; Vlim parameter
%Single Phase ZIP Load
%Author: Arun Suresh, University of North Carolina, Charlotte
%Iinj=((Pnom+jQnom)/Vmeas)'
function Iinj = InjectedCurrent(Vmeas,LoadType,Vnom,Pnom,Qnom,Vlim)
% Calculate Pl and Ql.
Kz=0;Ki=0;Kp=0;
Vk=(abs(Vmeas)/Vnom);%(Vmeas/Vnom)
switch LoadType  % 1 for Constant Z, 2 for Constant I and 3 for Constant P, 
    case 1
        Kz=1;
    case 2
        if Vk >= Vlim % convert to Constant Z load due to voltage violation
            Ki=1;
        else
            Kz=1;
        end
    case 3
        if Vk >= Vlim % convert to Constant Z load due to voltage violation
           Kp=1;
        else
            Kz=1;
        end          
 
end
Pl=Pnom *((Kz*Vk*Vk)+(Ki*Vk)+(Kp));
Ql=Qnom *((Kz*Vk*Vk)+(Ki*Vk)+(Kp));
% Net Injected Curent.
% j=sqrt(-1);
Iinj = conj((Pl+j*Ql)/Vmeas);
